simulink model "main"  (R2018a)
settings: Solver=VariableStepAuto  StartTime=0.0  StopTime=inf  RelTol=1e-3
libraries: aerolibutil x4, shared6dof x1, vrlib x1, aerolibanimutils x1
settings Model: Creator=PSere  LastModifiedBy=PSere

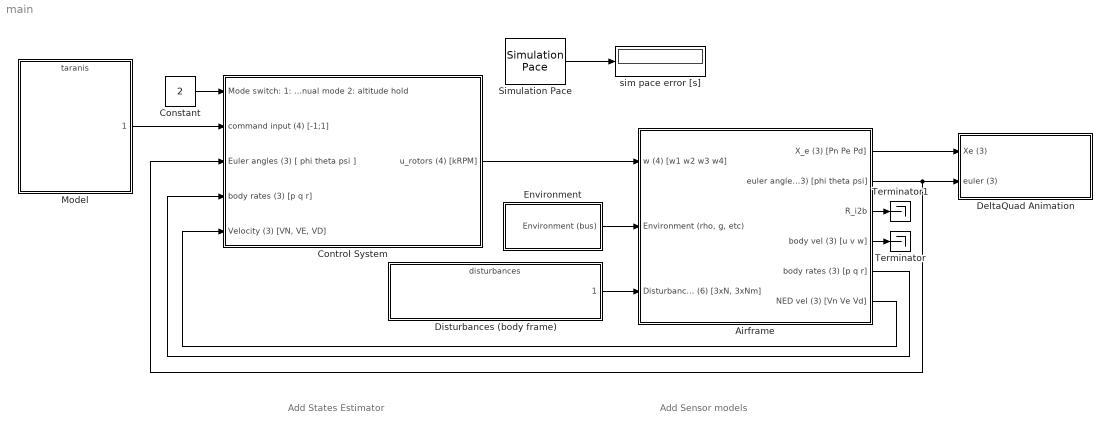
== system main ==
  note: Add Sensor models
  note: Add States Estimator
  Airframe : Subsystem
  Constant : Constant  Value=2
  Control System : Subsystem
  DeltaQuad Animation : Subsystem
  Disturbances (body frame) : ModelReference  ModelNameDialog=disturbances  SimulationMode=Normal  ModelReferenceVersion=1.13
  Environment : Subsystem
  Model : ModelReference  ModelNameDialog=taranis.mdl  SimulationMode=Normal  ModelReferenceVersion=1.8
  Simulation Pace : aerolibanimutils/Simulation Pace  SimulationPace=1  SleepMode=MATLAB Thread  OutputPaceError=on  SampleTime=1/30
  Terminator : Terminator
  Terminator1 : Terminator
  sim pace error [s] : Display
  wires:
  Model/1 -> Control System/2(command input (4) [-1;1])
  Control System/1(u_rotors (4) [kRPM]) -> Airframe/1(w (4) [w1 w2 w3 w4])
  Environment/1(Environment (bus)) -> Airframe/2("Environment (rho, g, etc)")
  Airframe/1(X_e (3) [Pn Pe Pd]) -> DeltaQuad Animation/1(Xe (3))
  Airframe/4(body vel (3) [u v w]) -> Terminator/1
  Airframe/2(euler angles (3) [phi theta psi]) -> Control System/3(Euler angles (3) [ phi theta psi ]), DeltaQuad Animation/2(euler (3))
  Airframe/5(body rates (3) [p q r]) -> Control System/4(body rates (3) [p q r])
  Airframe/3(R_i2b) -> Terminator1/1
  Constant/1 -> Control System/1(Mode switch: 1: manual mode 2: altitude hold)
  Airframe/6("NED vel (3) [Vn Ve Vd] ") -> Control System/5("Velocity (3) [VN, VE, VD]")
  Disturbances (body frame)/1 -> Airframe/3("Disturbances (6) [3xN, 3xNm]")
  Simulation Pace/1 -> sim pace error [s]/1

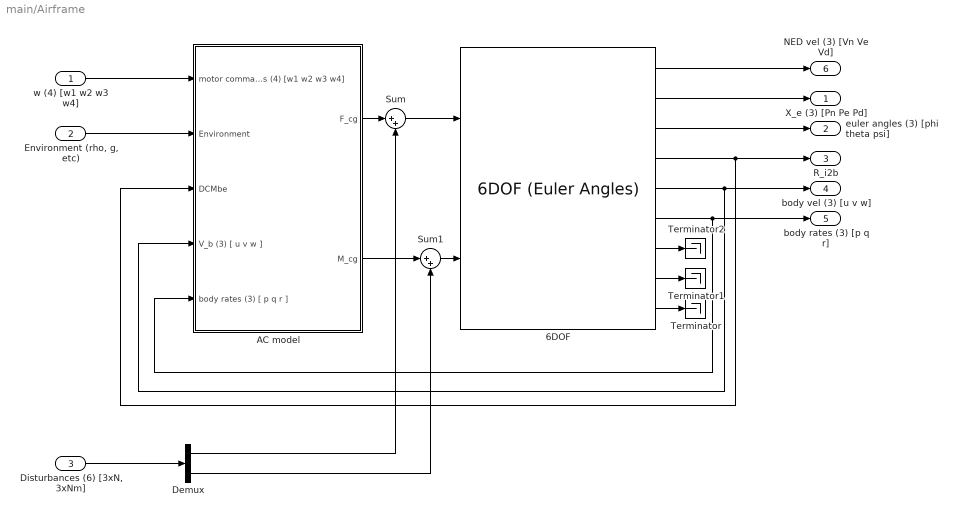
== system main/Airframe ==
  w (4) [w1 w2 w3 w4] : Inport
  "Environment (rho, g, etc)" : Inport  Port=2
  "Disturbances (6) [3xN, 3xNm]" : Inport  Port=3
  6DOF : shared6dof/6DOF (Euler Angles)  units=Metric (MKS)  mtype=Fixed  rep=Euler Angles  xme_0=[0,0,-10]  Vm_0=[0,0,0]  eul_0=[0,0,0]  pm_0=[0,0,0]  mass_0=5.0  mass_e=0.5  mass_f=2.0  inertia=|  inertia_e=eye(3)  inertia_f=2*eye(3)  k_quat=Vehicle.SixDOF.quatGain  vre_flag=on  abi_flag=on  aMode=aMode
      | [ 0.13, 0, -0.0015; 0, 0.0576, 0;
      |  -0.0015, 0, 0.3];
      settings: SourceProductBaseCode=AE
  AC model : Subsystem
  Demux : Demux  Outputs=[3, 3]
  Sum : Sum  Inputs=|++
  Sum1 : Sum  Inputs=|++
  Terminator : Terminator
  Terminator1 : Terminator
  Terminator2 : Terminator
  X_e (3) [Pn Pe Pd] : Outport
  euler angles (3) [phi theta psi] : Outport  Port=2
  R_i2b : Outport  Port=3
  body vel (3) [u v w] : Outport  Port=4
  body rates (3) [p q r] : Outport  Port=5
  "NED vel (3) [Vn Ve Vd] " : Outport  Port=6
  wires:
  6DOF/5 -> AC model/4(V_b (3) [ u v w ]), body vel (3) [u v w]/1
  6DOF/9 -> Terminator/1
  6DOF/8 -> Terminator1/1
  6DOF/7 -> Terminator2/1
  6DOF/1 -> "NED vel (3) [Vn Ve Vd] "/1
  6DOF/6 -> body rates (3) [p q r]/1, AC model/5(body rates (3) [ p q r ])
  "Environment (rho, g, etc)"/1 -> AC model/2(Environment)
  w (4) [w1 w2 w3 w4]/1 -> AC model/1(motor commands (4) [w1 w2 w3 w4])
  AC model/1(F_cg) -> Sum/1
  AC model/2(M_cg) -> Sum1/1
  6DOF/4 -> R_i2b/1, AC model/3(DCMbe)
  6DOF/2 -> X_e (3) [Pn Pe Pd]/1
  6DOF/3 -> euler angles (3) [phi theta psi]/1
  "Disturbances (6) [3xN, 3xNm]"/1 -> Demux/1
  Sum/1 -> 6DOF/1
  Sum1/1 -> 6DOF/2
  Demux/1 -> Sum/2
  Demux/2 -> Sum1/2

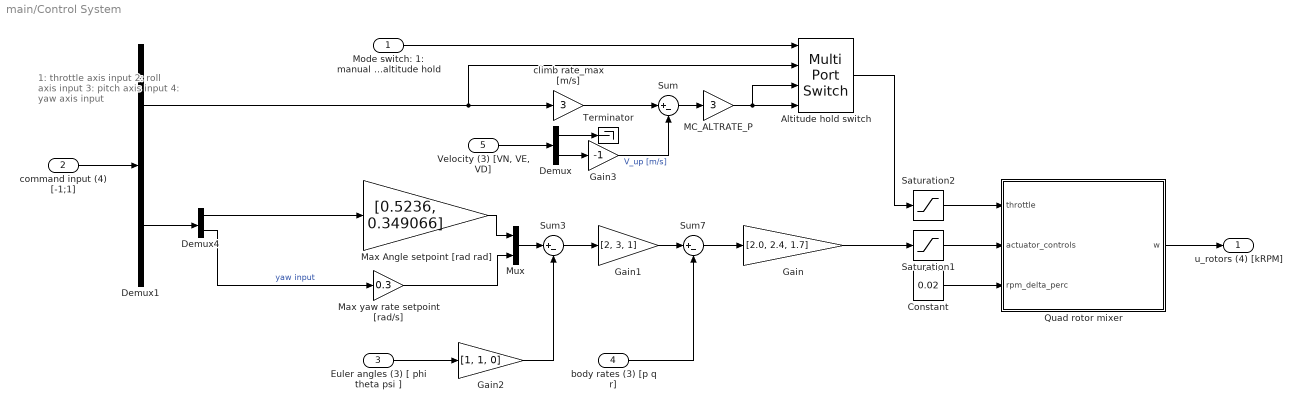
== system main/Control System ==
  note: 1: throttle axis input
      | 2: roll axis input
      | 3: pitch axis input
      | 4: yaw axis input
  Mode switch: 1: manual mode 2: altitude hold : Inport
  command input (4) [-1;1] : Inport  Port=2
  Euler angles (3) [ phi theta psi ] : Inport  Port=3
  body rates (3) [p q r] : Inport  Port=4
  "Velocity (3) [VN, VE, VD]" : Inport  Port=5
  Altitude hold switch : MultiPortSwitch
  Constant : Constant  Value=0.02
  Demux : Demux  Outputs=[2, 1]
  Demux1 : Demux  Outputs=[1 3]
  Demux4 : Demux  Outputs=[2,1]
  Gain : Gain  Gain=[2.0, 2.4, 1.7]
  Gain1 : Gain  Gain=[2, 3, 1]
  Gain2 : Gain  Gain=[1, 1, 0]
  Gain3 : Gain  Gain=-1
  MC_ALTRATE_P : Gain  Gain=3
  Max Angle setpoint [rad rad] : Gain  Gain=[0.5236, 0.349066]
  Max yaw rate setpoint [rad/s] : Gain  Gain=0.3
  Mux : Mux  Inputs=[2,1]
  Quad rotor mixer : MATLAB Function  TreatAsAtomicUnit=on
  Saturation1 : Saturate  UpperLimit=1  LowerLimit=-1
  Saturation2 : Saturate  UpperLimit=1  LowerLimit=-1
  Sum : Sum  Inputs=|+-
  Sum3 : Sum  Inputs=|+-
  Sum7 : Sum  Inputs=|+-
  Terminator : Terminator
  climb rate_max [m/s] : Gain  Gain=3
  u_rotors (4) [kRPM] : Outport
  wires:
  Quad rotor mixer/1(w) -> u_rotors (4) [kRPM]/1
  Constant/1 -> Quad rotor mixer/3(rpm_delta_perc)
  command input (4) [-1;1]/1 -> Demux1/1
  Saturation1/1 -> Quad rotor mixer/2(actuator_controls)
  Sum7/1 -> Gain/1
  body rates (3) [p q r]/1 -> Sum7/2
  Gain1/1 -> Sum7/1
  Gain/1 -> Saturation1/1
  Sum3/1 -> Gain1/1
  Gain2/1 -> Sum3/2
  Max Angle setpoint [rad rad]/1 -> Mux/1
  Demux1/2 -> Demux4/1
  Mode switch: 1: manual mode 2: altitude hold/1 -> Altitude hold switch/1
  Sum/1 -> MC_ALTRATE_P/1
  MC_ALTRATE_P/1 -> Altitude hold switch/4, Altitude hold switch/3
  Demux/1 -> Terminator/1
  Demux/2 -> Gain3/1
  Demux1/1 -> climb rate_max [m/s]/1, Altitude hold switch/2
  Altitude hold switch/1 -> Saturation2/1
  Saturation2/1 -> Quad rotor mixer/1(throttle)
  Gain3/1 -> Sum/2  "V_up [m/s]"
  climb rate_max [m/s]/1 -> Sum/1
  Demux4/1 -> Max Angle setpoint [rad rad]/1
  "Velocity (3) [VN, VE, VD]"/1 -> Demux/1
  Mux/1 -> Sum3/1
  Demux4/2 -> Max yaw rate setpoint [rad/s]/1  "yaw input"
  Max yaw rate setpoint [rad/s]/1 -> Mux/2
  Euler angles (3) [ phi theta psi ]/1 -> Gain2/1

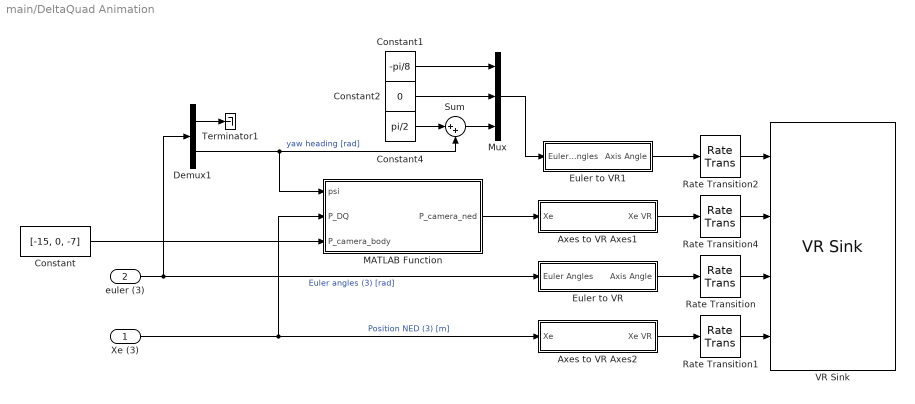
== system main/DeltaQuad Animation ==
  Xe (3) : Inport
  euler (3) : Inport  Port=2
  Axes to VR Axes1 : Subsystem
  Axes to VR Axes2 : Subsystem
  Constant : Constant  Value=[-15, 0, -7]
  Constant1 : Constant  Value=-pi/8
  Constant2 : Constant  Value=0
  Constant4 : Constant  Value=pi/2
  Demux1 : Demux  Outputs=[2 1]
  Euler to VR : Subsystem
  Euler to VR1 : Subsystem
  MATLAB Function : MATLAB Function  TreatAsAtomicUnit=on
  Mux : Mux  Inputs=3
  Rate Transition{,1..2,4} (4 alike) : RateTransition
  Sum : Sum  Inputs=|++
  Terminator1 : Terminator
  VR Sink : vrlib/VR Sink  InstantiateOnLoad=on  SampleTime=-1  ViewEnable=on  RemoteChange=off  RemoteView=off  FieldsWritten=Gimballed.orientation.4.1.1.double#Gimballed.position.3.1.1.double#DeltaQuad.rotation.4.1.1.double#DeltaQuad.translation.3.1.1.double  WorldFileName=animation\DQ_sim_simple.wrl  AutoView=off  VideoDimensions=[]  AllowVariableSize=off  FigureProperties="{'Position', 'Name', 'Viewpoint', 'CameraBound', 'CameraDirection', 'CameraPosition', 'CameraUpVector', 'ZoomFactor', 'Antialiasing', 'Headlight', 'Lighting', 'NavPanel', 'Sound', 'StatusBar', 'Stereo3D', 'Stereo3DCameraOffset', 'Stereo3DHIT', 'ToolBar', 'Textures', 'Transparency', 'Triad', 'Wireframe', 'NavZones', 'NavMode', 'NavSpeed', 'CaptureFileFormat', 'CaptureFileName', 'Record2DCompressMethod', 'Record2DCompressQuality', 'Record2D', 'Record2DFileName', 'Record2DFPS'; [5.5000000000000000e+01   1.2700000000000000e+02   9.1700000000000000e+02   6.5300000000000000e+02], '', 'Gimballed', 'on', [0.0000000000000000e+00   0.0000000000000000e+00  -1.0000000000000000e+00], [0.0000000000000000e+00   0.0000000000000000e+00   0.0000000000000000e+00], [0.0000000000000000e+00   1.0000000000000000e+00   0.0000000000000000e+00], [1.0000000000000000e+00], 'on', 'on', 'on', 'halfbar', 'on', 'on', 'off', [1.0000000149011612e-01], [0.0000000000000000e+00], 'on', 'on', 'on', 'none', 'off', 'off', 'fly', 'normal', 'tif', '%f_anim_%n.tif', 'auto', [7.5000000000000000e+01], 'off', '%f_anim_%n.avi', 'auto'}"
      settings: SourceProductBaseCode=VR
  wires:
  Euler to VR/1(Axis Angle) -> Rate Transition/1
  euler (3)/1 -> Euler to VR/1(Euler Angles), Demux1/1  "Euler angles (3) [rad]"
  Xe (3)/1 -> MATLAB Function/2(P_DQ), Axes to VR Axes2/1(Xe)  "Position NED (3) [m]"
  Axes to VR Axes2/1(Xe VR) -> Rate Transition1/1
  Rate Transition/1 -> VR Sink/3
  Rate Transition1/1 -> VR Sink/4
  Rate Transition4/1 -> VR Sink/2
  Rate Transition2/1 -> VR Sink/1
  Euler to VR1/1(Axis Angle) -> Rate Transition2/1
  Axes to VR Axes1/1(Xe VR) -> Rate Transition4/1
  MATLAB Function/1(P_camera_ned) -> Axes to VR Axes1/1(Xe)
  Constant/1 -> MATLAB Function/3(P_camera_body)
  Sum/1 -> Mux/3
  Demux1/2 -> MATLAB Function/1(psi), Sum/2  "yaw heading [rad]"
  Constant4/1 -> Sum/1
  Constant2/1 -> Mux/2
  Constant1/1 -> Mux/1
  Mux/1 -> Euler to VR1/1(Euler Angles)
  Demux1/1 -> Terminator1/1

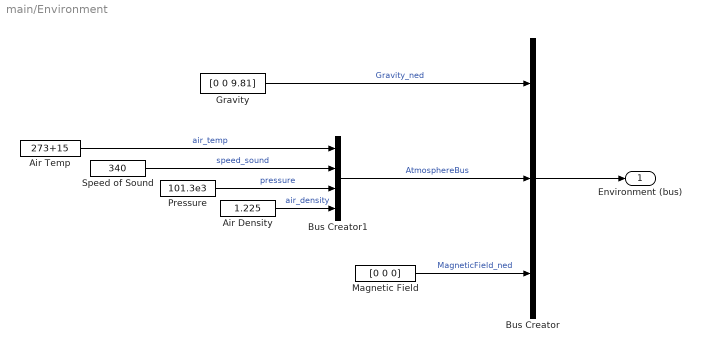
== system main/Environment ==
  Air Density : Constant  Value=1.225
  Air Temp : Constant  Value=273+15
  Bus Creator : BusCreator  Inputs=3
  Bus Creator1 : BusCreator  Inputs=4
  Gravity : Constant  Value=[0 0 9.81]
  Magnetic Field : Constant  Value=[0 0 0]
  Pressure : Constant  Value=101.3e3
  Speed of Sound : Constant  Value=340
  Environment (bus) : Outport
  wires:
  Air Temp/1 -> Bus Creator1/1  "air_temp"
  Magnetic Field/1 -> Bus Creator/3  "MagneticField_ned"
  Speed of Sound/1 -> Bus Creator1/2  "speed_sound"
  Gravity/1 -> Bus Creator/1  "Gravity_ned"
  Bus Creator1/1 -> Bus Creator/2  "AtmosphereBus"
  Bus Creator/1 -> Environment (bus)/1
  Air Density/1 -> Bus Creator1/4  "air_density"
  Pressure/1 -> Bus Creator1/3  "pressure"

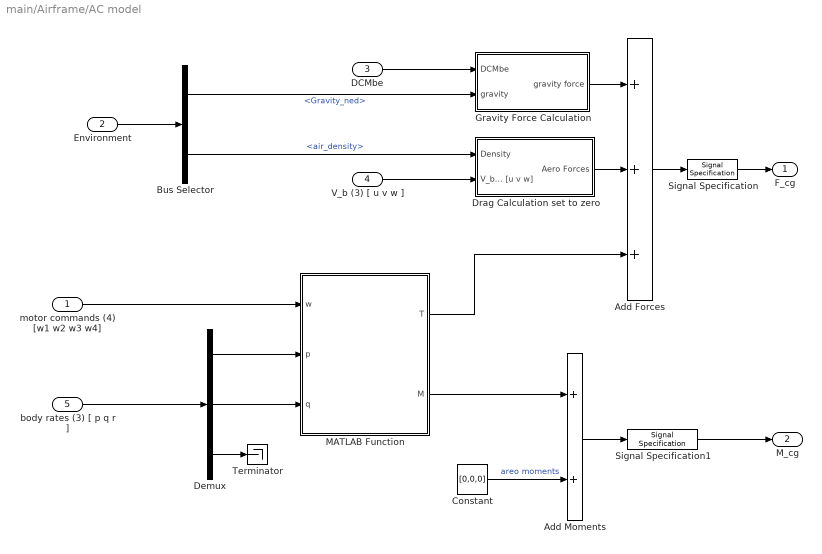
== system main/Airframe/AC model ==
  motor commands (4) [w1 w2 w3 w4] : Inport
  Environment : Inport  Port=2
  DCMbe : Inport  Port=3
  V_b (3) [ u v w ] : Inport  Port=4  Unit=m/s
  body rates (3) [ p q r ] : Inport  Port=5  Unit=rad/s
  Add Forces : Sum  Inputs=+++
  Add Moments : Sum
  Bus Selector : BusSelector  OutputSignals=Gravity_ned,AtmosphereBus.air_density
  Constant : Constant  Value=[0,0,0]
  Demux : Demux  Outputs=3
  Drag Calculation set to zero : Subsystem
  Gravity Force Calculation : Subsystem
  MATLAB Function : MATLAB Function  TreatAsAtomicUnit=on
  Signal Specification : SignalSpecification  Dimensions=3
  Signal Specification1 : SignalSpecification  Unit=N*m  Dimensions=3
  Terminator : Terminator
  F_cg : Outport  Unit=N
  M_cg : Outport  Port=2
  wires:
  Signal Specification/1 -> F_cg/1
  Bus Selector/1 -> Gravity Force Calculation/2(gravity)  "<Gravity_ned>"
  Environment/1 -> Bus Selector/1
  Bus Selector/2 -> Drag Calculation set to zero/1(Density)  "<air_density>"
  DCMbe/1 -> Gravity Force Calculation/1(DCMbe)
  V_b (3) [ u v w ]/1 -> Drag Calculation set to zero/2(V_body [u v w])
  Gravity Force Calculation/1(gravity force) -> Add Forces/1
  Drag Calculation set to zero/1(Aero Forces) -> Add Forces/2
  Add Forces/1 -> Signal Specification/1
  Add Moments/1 -> Signal Specification1/1
  MATLAB Function/1(T) -> Add Forces/3
  MATLAB Function/2(M) -> Add Moments/1
  Constant/1 -> Add Moments/2  "areo moments"
  Signal Specification1/1 -> M_cg/1
  Demux/2 -> MATLAB Function/3(q)
  Demux/1 -> MATLAB Function/2(p)
  motor commands (4) [w1 w2 w3 w4]/1 -> MATLAB Function/1(w)
  Demux/3 -> Terminator/1
  body rates (3) [ p q r ]/1 -> Demux/1

== system main/DeltaQuad Animation/Axes to VR Axes1 ==
  Xe : Inport
  Demux : Demux  Outputs=3
  Mux : Mux  Inputs=3
  rad-->deg1 : Gain  Gain=-1  SaturateOnIntegerOverflow=on  OutDataTypeStr=Inherit: Same as input  ParamDataTypeStr=Inherit: Same as input
  Xe VR : Outport
  wires:
  Xe/1 -> Demux/1
  Demux/1 -> Mux/1
  Demux/3 -> rad-->deg1/1
  Mux/1 -> Xe VR/1
  rad-->deg1/1 -> Mux/2
  Demux/2 -> Mux/3

== system main/DeltaQuad Animation/Axes to VR Axes2 ==
  Xe : Inport
  Demux : Demux  Outputs=3
  Mux : Mux  Inputs=3
  rad-->deg1 : Gain  Gain=-1  SaturateOnIntegerOverflow=on  OutDataTypeStr=Inherit: Same as input  ParamDataTypeStr=Inherit: Same as input
  Xe VR : Outport
  wires:
  Xe/1 -> Demux/1
  Demux/1 -> Mux/1
  Demux/3 -> rad-->deg1/1
  Mux/1 -> Xe VR/1
  rad-->deg1/1 -> Mux/2
  Demux/2 -> Mux/3

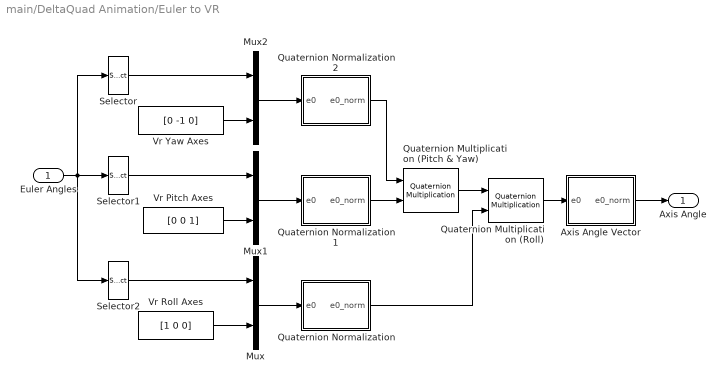
== system main/DeltaQuad Animation/Euler to VR ==
  Euler Angles : Inport
  Axis Angle Vector : Subsystem
  Mux : Mux  Inputs=2
  Mux1 : Mux  Inputs=2
  Mux2 : Mux  Inputs=2
  Quaternion Multiplication (Pitch & Yaw) : aerolibutil/Quaternion Multiplication
  Quaternion Multiplication (Roll) : aerolibutil/Quaternion Multiplication
  Quaternion Normalization : Subsystem
  Quaternion Normalization1 : Subsystem
  Quaternion Normalization2 : Subsystem
  Selector : Selector  InputPortWidth=3  IndexOptions=Index vector (dialog)  Indices=[3]  OutputSizes=1
  Selector1 : Selector  InputPortWidth=3  IndexOptions=Index vector (dialog)  Indices=[2]  OutputSizes=1
  Selector2 : Selector  InputPortWidth=3  IndexOptions=Index vector (dialog)  Indices=[1]  OutputSizes=1
  Vr Pitch Axes : Constant  Value=[0 0 1]
  Vr Roll Axes : Constant  Value=[1 0 0]
  Vr Yaw Axes : Constant  Value=[0 -1 0]
  Axis Angle : Outport
  wires:
  Quaternion Multiplication (Roll)/1 -> Axis Angle Vector/1(e0)
  Axis Angle Vector/1(e0_norm) -> Axis Angle/1
  Quaternion Normalization/1(e0_norm) -> Quaternion Multiplication (Roll)/2
  Quaternion Normalization2/1(e0_norm) -> Quaternion Multiplication (Pitch & Yaw)/1
  Quaternion Normalization1/1(e0_norm) -> Quaternion Multiplication (Pitch & Yaw)/2
  Mux2/1 -> Quaternion Normalization2/1(e0)
  Mux1/1 -> Quaternion Normalization1/1(e0)
  Mux/1 -> Quaternion Normalization/1(e0)
  Selector/1 -> Mux2/1
  Vr Yaw Axes/1 -> Mux2/2
  Selector1/1 -> Mux1/1
  Vr Pitch Axes/1 -> Mux1/2
  Selector2/1 -> Mux/1
  Vr Roll Axes/1 -> Mux/2
  Euler Angles/1 -> Selector2/1, Selector1/1, Selector/1
  Quaternion Multiplication (Pitch & Yaw)/1 -> Quaternion Multiplication (Roll)/1

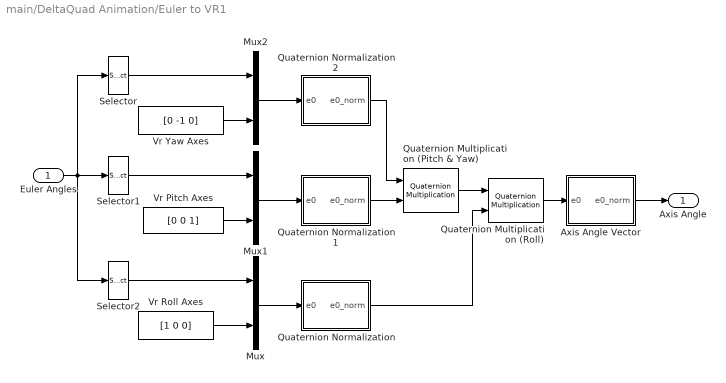
== system main/DeltaQuad Animation/Euler to VR1 ==
  Euler Angles : Inport
  Axis Angle Vector : Subsystem
  Mux : Mux  Inputs=2
  Mux1 : Mux  Inputs=2
  Mux2 : Mux  Inputs=2
  Quaternion Multiplication (Pitch & Yaw) : aerolibutil/Quaternion Multiplication
  Quaternion Multiplication (Roll) : aerolibutil/Quaternion Multiplication
  Quaternion Normalization : Subsystem
  Quaternion Normalization1 : Subsystem
  Quaternion Normalization2 : Subsystem
  Selector : Selector  InputPortWidth=3  IndexOptions=Index vector (dialog)  Indices=[3]  OutputSizes=1
  Selector1 : Selector  InputPortWidth=3  IndexOptions=Index vector (dialog)  Indices=[2]  OutputSizes=1
  Selector2 : Selector  InputPortWidth=3  IndexOptions=Index vector (dialog)  Indices=[1]  OutputSizes=1
  Vr Pitch Axes : Constant  Value=[0 0 1]
  Vr Roll Axes : Constant  Value=[1 0 0]
  Vr Yaw Axes : Constant  Value=[0 -1 0]
  Axis Angle : Outport
  wires:
  Quaternion Multiplication (Roll)/1 -> Axis Angle Vector/1(e0)
  Axis Angle Vector/1(e0_norm) -> Axis Angle/1
  Quaternion Normalization/1(e0_norm) -> Quaternion Multiplication (Roll)/2
  Quaternion Normalization2/1(e0_norm) -> Quaternion Multiplication (Pitch & Yaw)/1
  Quaternion Normalization1/1(e0_norm) -> Quaternion Multiplication (Pitch & Yaw)/2
  Mux2/1 -> Quaternion Normalization2/1(e0)
  Mux1/1 -> Quaternion Normalization1/1(e0)
  Mux/1 -> Quaternion Normalization/1(e0)
  Selector/1 -> Mux2/1
  Vr Yaw Axes/1 -> Mux2/2
  Selector1/1 -> Mux1/1
  Vr Pitch Axes/1 -> Mux1/2
  Selector2/1 -> Mux/1
  Vr Roll Axes/1 -> Mux/2
  Euler Angles/1 -> Selector2/1, Selector1/1, Selector/1
  Quaternion Multiplication (Pitch & Yaw)/1 -> Quaternion Multiplication (Roll)/1

== system main/Airframe/AC model/Drag Calculation set to zero ==
  Density : Inport  Unit=kg/m^3
  V_body [u v w] : Inport  Port=2  Unit=m/second
  Aero forces : MATLAB Function  TreatAsAtomicUnit=on
  Gain3 : Gain  Gain=-1
  Product : Product  RndMeth=Zero
  Sign : Signum  ZeroCross=off
  Aero Forces : Outport  Unit=N
  wires:
  Sign/1 -> Gain3/1  "direction vector"
  Gain3/1 -> Product/2
  Product/1 -> Aero Forces/1  "Aero Forces"
  V_body [u v w]/1 -> Aero forces/2(V), Sign/1
  Density/1 -> Aero forces/1(rho)
  Aero forces/1(F) -> Product/1

== system main/Airframe/AC model/Gravity Force Calculation ==
  DCMbe : Inport
  gravity : Inport  Port=2  Unit=m/s^2
  Product : Product  Multiplication=Matrix(*)
  mass [kg] : Gain  Gain=5.0
  gravity force : Outport  Unit=N
  wires:
  gravity/1 -> mass [kg]/1
  mass [kg]/1 -> Product/2  "gravity force NED"
  Product/1 -> gravity force/1
  DCMbe/1 -> Product/1

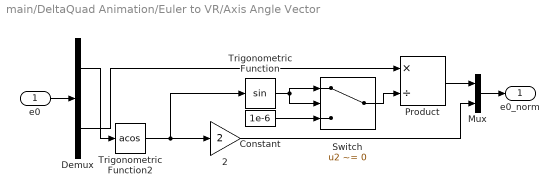
== system main/DeltaQuad Animation/Euler to VR/Axis Angle Vector ==
  e0 : Inport
  2 : Gain  Gain=2  SaturateOnIntegerOverflow=on  OutDataTypeStr=Inherit: Same as input  ParamDataTypeStr=Inherit: Same as input
  Constant : Constant  Value=1e-6
  Demux : Demux  Outputs=[1 3 ]
  Mux : Mux  Inputs=2
  Product : Product  Inputs=*/  SaturateOnIntegerOverflow=on  InputSameDT=on  OutDataTypeStr=Inherit: Same as first input
  Switch : Switch  Criteria=u2 ~= 0
  Trigonometric Function : Trigonometry
  Trigonometric Function2 : Trigonometry  Operator=acos
  e0_norm : Outport
  wires:
  Demux/1 -> Trigonometric Function2/1
  Demux/2 -> Product/1
  Mux/1 -> e0_norm/1
  Product/1 -> Mux/1
  2/1 -> Mux/2
  Trigonometric Function/1 -> Switch/1, Switch/2
  Trigonometric Function2/1 -> Trigonometric Function/1, 2/1
  e0/1 -> Demux/1
  Constant/1 -> Switch/3
  Switch/1 -> Product/2

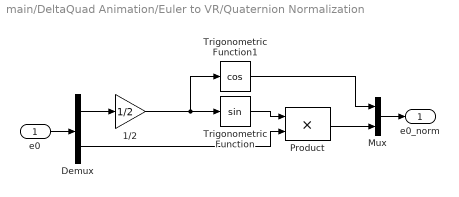
== system main/DeltaQuad Animation/Euler to VR/Quaternion Normalization ==
  e0 : Inport
  1/2 : Gain  Gain=1/2  SaturateOnIntegerOverflow=on  OutDataTypeStr=Inherit: Same as input  ParamDataTypeStr=Inherit: Same as input
  Demux : Demux  Outputs=[1 3]
  Mux : Mux  Inputs=2
  Product : Product  SaturateOnIntegerOverflow=on  InputSameDT=on  OutDataTypeStr=Inherit: Same as first input
  Trigonometric Function : Trigonometry
  Trigonometric Function1 : Trigonometry  Operator=cos
  e0_norm : Outport
  wires:
  Trigonometric Function1/1 -> Mux/1
  Demux/2 -> Product/2
  Demux/1 -> 1/2/1
  Mux/1 -> e0_norm/1
  Product/1 -> Mux/2
  Trigonometric Function/1 -> Product/1
  1/2/1 -> Trigonometric Function1/1, Trigonometric Function/1
  e0/1 -> Demux/1

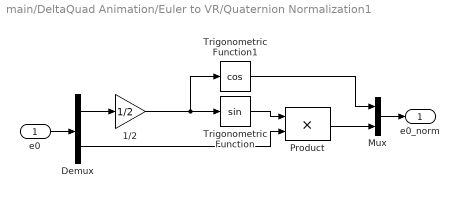
== system main/DeltaQuad Animation/Euler to VR/Quaternion Normalization1 ==
  e0 : Inport
  1/2 : Gain  Gain=1/2  SaturateOnIntegerOverflow=on  OutDataTypeStr=Inherit: Same as input  ParamDataTypeStr=Inherit: Same as input
  Demux : Demux  Outputs=[1 3]
  Mux : Mux  Inputs=2
  Product : Product  SaturateOnIntegerOverflow=on  InputSameDT=on  OutDataTypeStr=Inherit: Same as first input
  Trigonometric Function : Trigonometry
  Trigonometric Function1 : Trigonometry  Operator=cos
  e0_norm : Outport
  wires:
  e0/1 -> Demux/1
  1/2/1 -> Trigonometric Function/1, Trigonometric Function1/1
  Trigonometric Function/1 -> Product/1
  Product/1 -> Mux/2
  Mux/1 -> e0_norm/1
  Demux/1 -> 1/2/1
  Demux/2 -> Product/2
  Trigonometric Function1/1 -> Mux/1

== system main/DeltaQuad Animation/Euler to VR/Quaternion Normalization2 ==
  e0 : Inport
  1/2 : Gain  Gain=1/2  SaturateOnIntegerOverflow=on  OutDataTypeStr=Inherit: Same as input  ParamDataTypeStr=Inherit: Same as input
  Demux : Demux  Outputs=[1 3]
  Mux : Mux  Inputs=2
  Product : Product  SaturateOnIntegerOverflow=on  InputSameDT=on  OutDataTypeStr=Inherit: Same as first input
  Trigonometric Function : Trigonometry
  Trigonometric Function1 : Trigonometry  Operator=cos
  e0_norm : Outport
  wires:
  Trigonometric Function1/1 -> Mux/1
  Demux/2 -> Product/2
  Demux/1 -> 1/2/1
  Mux/1 -> e0_norm/1
  Product/1 -> Mux/2
  Trigonometric Function/1 -> Product/1
  1/2/1 -> Trigonometric Function1/1, Trigonometric Function/1
  e0/1 -> Demux/1

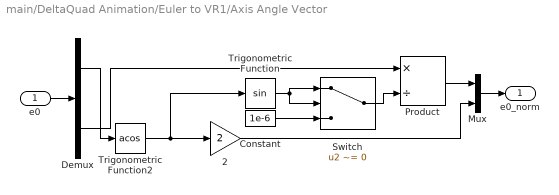
== system main/DeltaQuad Animation/Euler to VR1/Axis Angle Vector ==
  e0 : Inport
  2 : Gain  Gain=2  SaturateOnIntegerOverflow=on  OutDataTypeStr=Inherit: Same as input  ParamDataTypeStr=Inherit: Same as input
  Constant : Constant  Value=1e-6
  Demux : Demux  Outputs=[1 3 ]
  Mux : Mux  Inputs=2
  Product : Product  Inputs=*/  SaturateOnIntegerOverflow=on  InputSameDT=on  OutDataTypeStr=Inherit: Same as first input
  Switch : Switch  Criteria=u2 ~= 0
  Trigonometric Function : Trigonometry
  Trigonometric Function2 : Trigonometry  Operator=acos
  e0_norm : Outport
  wires:
  Demux/1 -> Trigonometric Function2/1
  Demux/2 -> Product/1
  Mux/1 -> e0_norm/1
  Product/1 -> Mux/1
  2/1 -> Mux/2
  Trigonometric Function/1 -> Switch/1, Switch/2
  Trigonometric Function2/1 -> Trigonometric Function/1, 2/1
  e0/1 -> Demux/1
  Constant/1 -> Switch/3
  Switch/1 -> Product/2

== system main/DeltaQuad Animation/Euler to VR1/Quaternion Normalization ==
  e0 : Inport
  1/2 : Gain  Gain=1/2  SaturateOnIntegerOverflow=on  OutDataTypeStr=Inherit: Same as input  ParamDataTypeStr=Inherit: Same as input
  Demux : Demux  Outputs=[1 3]
  Mux : Mux  Inputs=2
  Product : Product  SaturateOnIntegerOverflow=on  InputSameDT=on  OutDataTypeStr=Inherit: Same as first input
  Trigonometric Function : Trigonometry
  Trigonometric Function1 : Trigonometry  Operator=cos
  e0_norm : Outport
  wires:
  Trigonometric Function1/1 -> Mux/1
  Demux/2 -> Product/2
  Demux/1 -> 1/2/1
  Mux/1 -> e0_norm/1
  Product/1 -> Mux/2
  Trigonometric Function/1 -> Product/1
  1/2/1 -> Trigonometric Function1/1, Trigonometric Function/1
  e0/1 -> Demux/1

== system main/DeltaQuad Animation/Euler to VR1/Quaternion Normalization1 ==
  e0 : Inport
  1/2 : Gain  Gain=1/2  SaturateOnIntegerOverflow=on  OutDataTypeStr=Inherit: Same as input  ParamDataTypeStr=Inherit: Same as input
  Demux : Demux  Outputs=[1 3]
  Mux : Mux  Inputs=2
  Product : Product  SaturateOnIntegerOverflow=on  InputSameDT=on  OutDataTypeStr=Inherit: Same as first input
  Trigonometric Function : Trigonometry
  Trigonometric Function1 : Trigonometry  Operator=cos
  e0_norm : Outport
  wires:
  e0/1 -> Demux/1
  1/2/1 -> Trigonometric Function/1, Trigonometric Function1/1
  Trigonometric Function/1 -> Product/1
  Product/1 -> Mux/2
  Mux/1 -> e0_norm/1
  Demux/1 -> 1/2/1
  Demux/2 -> Product/2
  Trigonometric Function1/1 -> Mux/1

== system main/DeltaQuad Animation/Euler to VR1/Quaternion Normalization2 ==
  e0 : Inport
  1/2 : Gain  Gain=1/2  SaturateOnIntegerOverflow=on  OutDataTypeStr=Inherit: Same as input  ParamDataTypeStr=Inherit: Same as input
  Demux : Demux  Outputs=[1 3]
  Mux : Mux  Inputs=2
  Product : Product  SaturateOnIntegerOverflow=on  InputSameDT=on  OutDataTypeStr=Inherit: Same as first input
  Trigonometric Function : Trigonometry
  Trigonometric Function1 : Trigonometry  Operator=cos
  e0_norm : Outport
  wires:
  Trigonometric Function1/1 -> Mux/1
  Demux/2 -> Product/2
  Demux/1 -> 1/2/1
  Mux/1 -> e0_norm/1
  Product/1 -> Mux/2
  Trigonometric Function/1 -> Product/1
  1/2/1 -> Trigonometric Function1/1, Trigonometric Function/1
  e0/1 -> Demux/1

== matlab function main/Control System/Quad rotor mixer ==
  data: throttle input; w output; actuator_controls input; rpm_delta_perc input
function w   = fcn(throttle, actuator_controls, rpm_delta_perc)
%% INPUTS: 
% actuator controls: all range from -1 to 1
% 1: roll axis; 
% 2: pitch axis;
% 3: yaw axis;
% OUTPUT:
% w: 4 by 1 vector:
%       w(1): front right
%       w(2): front left
%       w(3): rear  left
%       w(4): rear  right
% Scale throttle to rpm:
throttle = 1 * (throttle + 1);          % -1 -> 0; +1 -> 2;  

%% Control signal deltas
% Scale input signals  
w = throttle * ones(4, 1); % Throttle scales all of them
w  = w + [ -1;  1;  1;  -1]   * rpm_delta_perc * actuator_controls(1);   
w  = w + [  1;  1; -1;  -1]   * rpm_delta_perc * actuator_controls(2);   
w  = w + [  1; -1;  1;  -1]   * rpm_delta_perc * actuator_controls(3);     
end

== matlab function main/Airframe/AC model/Drag Calculation set to zero/Aero forces ==
  data: rho input; V input; F output
function F = aero(rho, V)
%% INPUTS:
% rho:  density                              [kg/m3]
% V:    body velocities wrt air [ub, vb, wb] [m/s]
%TAS = norm(V);
%alpha = atan(V(3)/V(1));

%% DQ Parameters:
%S = 1.0;
%b = 1.9;

%e = 0.9;
%AR = b^2/S;
%qS = 0.5*rho*TAS^2*S;

%% Aerodynamic coefficients:
%Within 20 degree region we generate lift:
% 
% CL_0        = 0.0;
% CD_0        = 0.02;
% if abs(alpha*180/pi) < 10
%     CL_alpha = 1.1471;
%     
%     CL = CL_0 + CL_alpha * alpha;
%     CD = CD_0 + CL^2 / (pi*AR*e);
%     CY = 0;
%     
%     % Rotate the coordinate frame around Y-axis with alpha to get body axes 
%     F_liftdrag = [cos(alpha)    0   -sin(alpha);
%                   0             1   0;
%                   sin(alpha)    0   cos(alpha)]*[qS * CD; 
%                                                  qS * CY; 
%                                                  qS * CL];
%                                              
%                  
% else
% 
%     F_liftdrag = [0;0;0];
% end
%
% F_liftdrag = [0;0;0];
% 
% S = 1.0;
% 
% CD_X = 0.1;
% CD_Y = 0.1;
% CD_Z = 0.2;
% 
% F = [0.5 * rho * S * V(1)^2 * CD_X;
%      0.5 * rho * S * V(2)^2 * CD_Y;
%      0.5 * rho * S * V(3)^2 * CD_Z] + F_liftdrag;


 F = [0;
      0;
      0];

end

% Moments:
% %% Roll pitch and yaw moments as a function of alpha and beta:
% 
% Cl = Cl_beta  * beta;
% Cm = Cm_0 + Cm_alpha * alpha;
% Cn = Cn_beta  * beta;
% 
% Ma = [  b * qS * Cl; 
%         c * qS * Cm; 
%         b * qS * Cn];

== matlab function main/Airframe/AC model/MATLAB Function ==
  data: w input; T output; M output; p input; q input
function [T, M] = motor_model(w, p, q)
%% Deltaquad Parameters:
      
Irzz    = 0.05;                            % rotor inertia [kgm2]
dx      = 0.35;                            % position of rotors x
dy      = 0.35;                            % position of rotors y
k1      = 12.2625;                         % N / kRPM^2
k2      = 4.2;                             % Nm / kRPM^2

if length(w) ~= 4
    error('control vector wrong size')
end

%% Thrust and Moments:
% 1) Total Thrust body axis
T = [0; 0; -k1 * sum(w.^2)];

% 2) Mc: Conrol moments:
Mc = [-dy*k1, dy*k1,  dy*k1, -dy*k1;
       dx*k1, dx*k1, -dx*k1, -dx*k1;
       k2,    -k2,    k2,      -k2]*w.^2;
   
% 3) Mr: Gyro moments:
Mr = [ Irzz*q, -Irzz*q,  Irzz*q, -Irzz*q;
      -Irzz*p,  Irzz*p, -Irzz*p,  Irzz*p;
            0,       0,       0,       0]*w;

M = Mc - Mr;

== matlab function main/DeltaQuad Animation/MATLAB Function ==
  data: psi input; P_DQ input; P_camera_ned output; P_camera_body input
function P_camera_ned  = fcn(psi, P_DQ, P_camera_body)
R_b2i_phi = transpose([cos(psi), sin(psi),    0; -sin(psi), cos(psi),   0; 0, 0, 1]);
P_camera_ned = [P_DQ(1);P_DQ(2);P_DQ(3)] + R_b2i_phi * [P_camera_body(1);P_camera_body(2);P_camera_body(3)];
